simulink model "EarlyReturn5_2018a"  (R2018a)
settings: Solver=VariableStepAuto  StartTime=0.0  StopTime=0.1  RelTol=1e-3
settings Model: Creator=BEAR  LastModifiedBy=bzhan

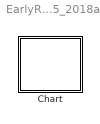
== system EarlyReturn5_2018a ==
  Chart : Stateflow chart  TreatAsAtomicUnit=on

== stateflow chart EarlyReturn5_2018a/Chart ==
  state A
    en: f("en_A")
    ex: f("ex_A")
    state A1
      en: f("en_A1")
      ex: f("ex_A1")
    state A2
      en: f("en_A2")
      ex: f("ex_A2")
    (default) -> A1
    A1 -> A2 : /{E;f("ta")}
  state B
    en: f("en_B")
    ex: f("ex_B")
  (default) -> A
  A -> B : E
  data: s function_input
  events: E local FUNCTION_CALL_EVENT
  function f(s):
    | function f(s)
    |   fprintf(s+"\n");
